simulink model "moveRobot"  (R2015b)
settings: Solver=FixedStepDiscrete  StartTime=0.0  StopTime=20  FixedStep=1  RelTol=1e-3
libraries: canmsglib x3, speedgoatlib_IO601 x3, slrtlib x1
settings Model: Creator=1SMARTe  LastModifiedBy=1SMARTe
settings SolverCC: EnableConcurrentExecution=on
settings OptimizationCC: BlockReduction=off  OptimizeBlockIOStorage=off  BufferReuse=off  GlobalBufferReuse=off  ExpressionFolding=off  LocalBlockOutputs=off
settings HardwareCC: ProdBitPerPointer=32  ProdLargestAtomicFloat=None  ProdWordSize=32  ProdLongLongMode=on  ProdHWDeviceType=Generic->32-bit x86 compatible
settings RTWCC: SystemTargetFile=slrt.tlc  TemplateMakefile=slrt_default_tmf  Description=Simulink Real-Time  RTWCompilerOptimization=on

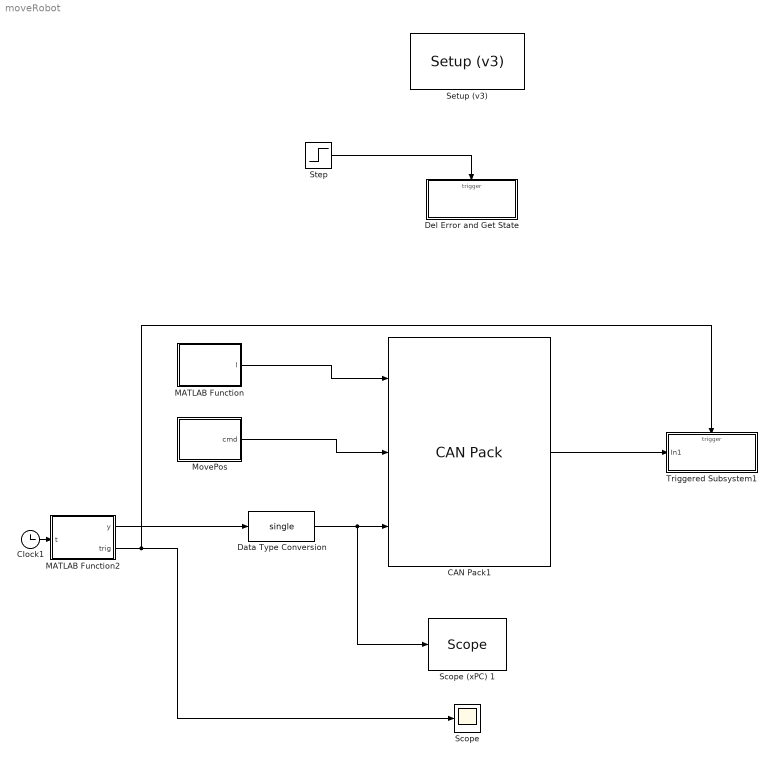
== system moveRobot ==
  CAN Pack1 : canmsglib/CAN Pack  MsgList=(none)  MsgName=MovePos  MsgIDType=Standard (11-bit identifier)  MsgIdentifier=1283  MsgLength=6  SignalInfo=Signal1$0$8$1$2$1$0$1$0$-Inf$Inf$#Signal2$8$8$1$2$1$0$1$0$-Inf$Inf$#Signal3$16$32$1$1$1$0$1$0$-Inf$Inf$#  NSignals=3  StartBits=str2num('[int32(0);int32(8);int32(16)]')  SignalSizes=str2num('[int32(8);int32(8);int32(32)]')  ByteOrders=str2num('[int32(1);int32(1);int32(1)]')  DataTypes=str2num('[int32(2);int32(2);int32(1)]')  MultiplexTypes=str2num('[int32(1);int32(1);int32(1)]')  MultiplexValues=str2num('[double(0);double(0);double(0)]')  Factors=str2num('[double(1);double(1);double(1)]')  Offsets=str2num('[double(0);double(0);double(0)]')  Minimums=str2num('[double(-Inf);double(-Inf);double(-Inf)]')  Maximums=str2num('[double(Inf);double(Inf);double(Inf)]')  Remote=off
      settings: DataFormat=manually specified signals
  Clock1 : Clock
  Data Type Conversion : DataTypeConversion  OutDataTypeStr=single
  Del Error and Get State : Subsystem  TreatAsAtomicUnit=on
  MATLAB Function : MATLAB Function  TreatAsAtomicUnit=on
  MATLAB Function2 : MATLAB Function  TreatAsAtomicUnit=on
  MovePos : MATLAB Function  TreatAsAtomicUnit=on
  Scope : Scope
  Scope (xPC) 1 : slrtlib/Displays and Logging/Scope   scopeno=1  scopetype=Target  autostart=on  viewmode=Numerical  formatstr='%15.6f'  grid=on  ylimits=[0,0]  nosamples=250  noprepostsamples=0  interleave=1  triggermode=Signal triggering  triggersignal=1  trigsignalfromport=off  triggerlevel=0.0  triggerslope=Rising  triggerscope=1  triggersample=0  filename=data.dat  mode=Lazy  writesize=512  autorestart=off  dynamicfilemode=off  maxwritefilesize=512*1024^2
  Setup (v3) : speedgoatlib_IO601/Setup (v3)  id=1  can1enable=on  can1bus=Highspeed  can1Baudrate=500 kBaud  can1UserBR=[1,1,5,2]  stdAcc1=[0,0,0,0]  extAcc1=[0,0,0,0]  can2enable=on  can2bus=Highspeed  can2Baudrate=500 kBaud  can2UserBR=[1,1,5,2]  stdAcc2=[0,0,0,0]  extAcc2=[0,0,0,0]  pciSlot=-1
  Step : Step  Time=2  SampleTime=0
  Triggered Subsystem1 : Subsystem  TreatAsAtomicUnit=on
  wires:
  MATLAB Function/1(l) -> CAN Pack1/1
  MovePos/1(cmd) -> CAN Pack1/2
  MATLAB Function2/1(y) -> Data Type Conversion/1
  Clock1/1 -> MATLAB Function2/1(t)
  Step/1 -> Del Error and Get State/Trigger
  CAN Pack1/1 -> Triggered Subsystem1/1(In1)
  MATLAB Function2/2(trig) -> Scope/1, Triggered Subsystem1/Trigger
  Data Type Conversion/1 -> Scope (xPC) 1/1, CAN Pack1/3

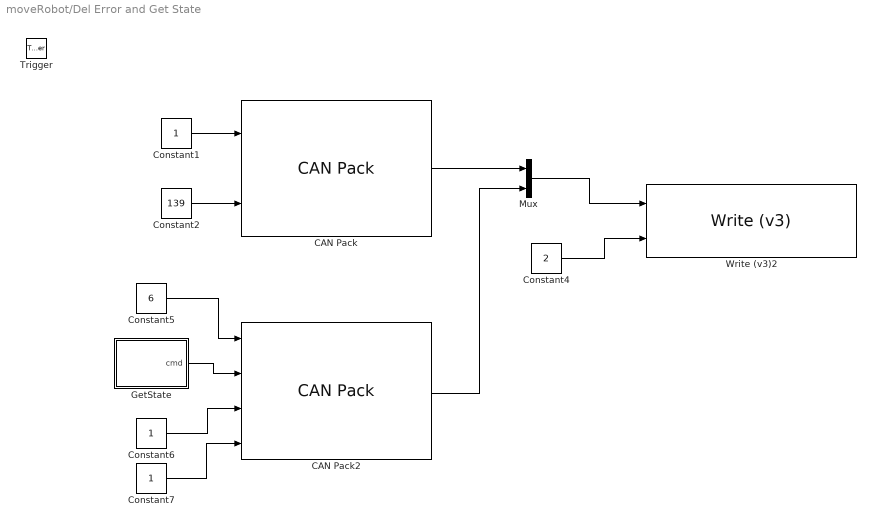
== system moveRobot/Del Error and Get State ==
  Trigger : TriggerPort
  CAN Pack : canmsglib/CAN Pack  MsgList=(none)  MsgName=QuitError  MsgIDType=Standard (11-bit identifier)  MsgIdentifier=1283  MsgLength=2  SignalInfo=Signal1$0$8$1$2$1$0$1$0$-Inf$Inf$#Signal2$8$8$1$2$1$0$1$0$-Inf$Inf$#  NSignals=2  StartBits=str2num('[int32(0);int32(8)]')  SignalSizes=str2num('[int32(8);int32(8)]')  ByteOrders=str2num('[int32(1);int32(1)]')  DataTypes=str2num('[int32(2);int32(2)]')  MultiplexTypes=str2num('[int32(1);int32(1)]')  MultiplexValues=str2num('[double(0);double(0)]')  Factors=str2num('[double(1);double(1)]')  Offsets=str2num('[double(0);double(0)]')  Minimums=str2num('[double(-Inf);double(-Inf)]')  Maximums=str2num('[double(Inf);double(Inf)]')  Remote=off
      settings: DataFormat=manually specified signals
  CAN Pack2 : canmsglib/CAN Pack  MsgList=(none)  MsgName=GetState  MsgIDType=Standard (11-bit identifier)  MsgIdentifier=1283  MsgLength=7  SignalInfo=Signal1$0$8$1$2$1$0$1$0$-Inf$Inf$#Signal2$8$8$1$2$1$0$1$0$-Inf$Inf$#time$16$32$1$2$1$0$1$0$-Inf$Inf$#mode$48$8$1$2$1$0$1$0$-Inf$Inf$#  NSignals=4  StartBits=str2num('[int32(0);int32(8);int32(16);int32(48)]')  SignalSizes=str2num('[int32(8);int32(8);int32(32);int32(8)]')  ByteOrders=str2num('[int32(1);int32(1);int32(1);int32(1)]')  DataTypes=str2num('[int32(2);int32(2);int32(2);int32(2)]')  MultiplexTypes=str2num('[int32(1);int32(1);int32(1);int32(1)]')  MultiplexValues=str2num('[double(0);double(0);double(0);double(0)]')  Factors=str2num('[double(1);double(1);double(1);double(1)]')  Offsets=str2num('[double(0);double(0);double(0);double(0)]')  Minimums=str2num('[double(-Inf);double(-Inf);double(-Inf);double(-Inf)]')  Maximums=str2num('[double(Inf);double(Inf);double(Inf);double(Inf)]')  Remote=off
      settings: DataFormat=manually specified signals
  Constant1 : Constant
  Constant2 : Constant  Value=139
  Constant4 : Constant  Value=2
  Constant5 : Constant  Value=6
  Constant6 : Constant
  Constant7 : Constant
  GetState : MATLAB Function  TreatAsAtomicUnit=on
  Mux : Mux  Inputs=2
  Write (v3)2 : speedgoatlib_IO601/Write (v3)  Priority=1  id=1  sampletime=-1  pciSlot=-1  inputType=CAN_MESSAGE plus count  port=1  maxMsg=2  status=off  init=[]  term=[]
  wires:
  Constant2/1 -> CAN Pack/2
  Constant1/1 -> CAN Pack/1
  Constant6/1 -> CAN Pack2/3
  CAN Pack2/1 -> Mux/2
  Constant7/1 -> CAN Pack2/4
  Constant5/1 -> CAN Pack2/1
  GetState/1(cmd) -> CAN Pack2/2
  CAN Pack/1 -> Mux/1
  Constant4/1 -> Write (v3)2/2
  Mux/1 -> Write (v3)2/1

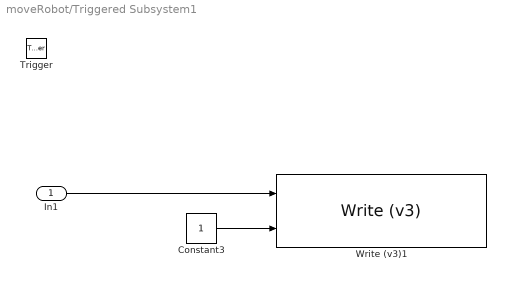
== system moveRobot/Triggered Subsystem1 ==
  In1 : Inport
  Trigger : TriggerPort
  Constant3 : Constant
  Write (v3)1 : speedgoatlib_IO601/Write (v3)  Priority=1  id=1  sampletime=-1  pciSlot=-1  inputType=CAN_MESSAGE plus count  port=1  maxMsg=1  status=off  init=[]  term=[]
  wires:
  Constant3/1 -> Write (v3)1/2
  In1/1 -> Write (v3)1/1

== matlab function moveRobot/MovePos ==
  data: cmd output
function cmd = fcn()
%#codegen

cmd = hex2dec('B0');

== matlab function moveRobot/MATLAB Function ==
  data: l output
function l = fcn()
%#codegen

l = hex2dec('05');

== matlab function moveRobot/MATLAB Function2 ==
  data: y output; t input; trig output
function [y,trig] = fcn(t)
%#codegen
trig = 0;
y=0;
if t == 5
    trig = 1;
    y = 90000;
end
if t>5
    trig = 0;
end
if t>15
    trig = 1;
    y = 0;
end

== matlab function moveRobot/Del Error and Get State/GetState ==
  data: cmd output
function cmd = fcn()
%#codegen

cmd = hex2dec('95');
